simulink model "SegwayControlledNot0"  (R2019a)
settings: Solver=VariableStepAuto  StartTime=0.0  StopTime=10.0  RelTol=1e-3
undefined symbols (not defined in the file): A, B, C, D, K, Kr, TargetPP2, X0ToPosAngle
settings Model: Creator=Huynh  LastModifiedBy=Huynh

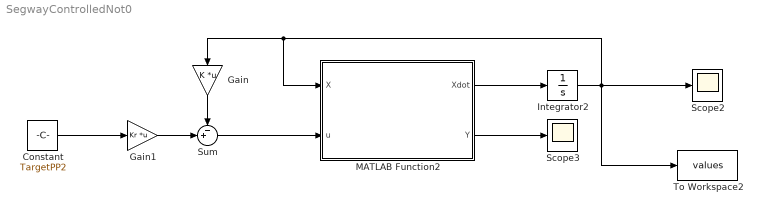
== system SegwayControlledNot0 ==
  Constant : Constant  Value=TargetPP2
  Gain : Gain  Gain=K  Multiplication=Matrix(K*u)
  Gain1 : Gain  Gain=Kr  Multiplication=Matrix(K*u)
  Integrator2 : Integrator  InitialCondition=X0ToPosAngle
  MATLAB Function2 : MATLAB Function  TreatAsAtomicUnit=on
  Scope2 : Scope
  Scope3 : Scope
  Sum : Sum  Inputs=-+|
  To Workspace2 : ToWorkspace  VariableName=values  SampleTime=-1
  wires:
  Gain/1 -> Sum/1
  MATLAB Function2/1(Xdot) -> Integrator2/1
  Integrator2/1 -> Gain/1, MATLAB Function2/1(X), To Workspace2/1, Scope2/1
  MATLAB Function2/2(Y) -> Scope3/1
  Sum/1 -> MATLAB Function2/2(u)
  Gain1/1 -> Sum/2
  Constant/1 -> Gain1/1

== matlab function SegwayControlledNot0/MATLAB Function2 ==
  data: X input; Xdot output; A parameter; B parameter; C parameter; D parameter; Y output; u input
function [Xdot, Y] = LinearZeroSegway(X, A, B, C, D, u)
Xdot = A * X + B * u;
Y = C*X + D*u;
end
